simulink model "System_R2"  (R2018b)
settings: Solver=VariableStepAuto  StartTime=0.0  StopTime=5  RelTol=1e-3
libraries: dspsrcs4 x2, simulink x2
settings Model: Creator=Whtest  LastModifiedBy=Whtest

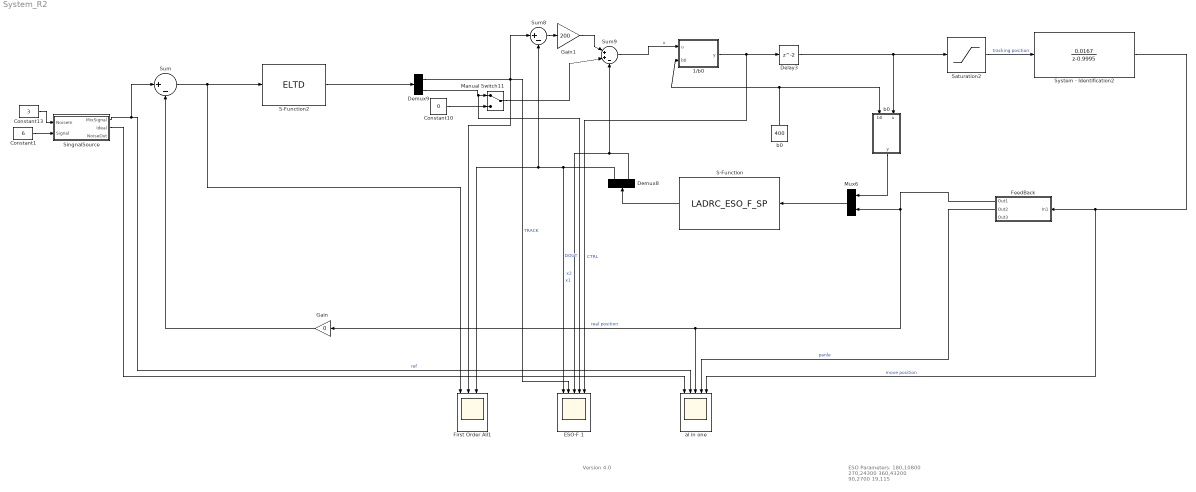
== system System_R2 ==
  note: ESO Parameters:
      | 180,10800
      | 270,24300
      | 360,43200
      | 90,2700
      | 19,115
  note: Version 4.0
  " b0" : MATLAB Function  TreatAsAtomicUnit=on
  1/b0 : MATLAB Function  TreatAsAtomicUnit=on
  Constant1 : Constant  Value=6
  Constant10 : Constant  Value=0
  Constant13 : Constant  Value=3
  Delay3 : Delay
  Demux8 : Demux  Outputs=2
  Demux9 : Demux  Outputs=2
  ESO-F 1 : Scope  NumInputPorts=5
  FeedBack : Subsystem
  First Order All1 : Scope  NumInputPorts=4
  Gain : Gain  Gain=0
  Gain1 : Gain  Gain=200
  Manual Switch11 : ManualSwitch
  Mux6 : Mux  Inputs=2
  S-Function : S-Function  FunctionName=LADRC_ESO_F_SP  Parameters=124  SFunctionDeploymentMode=off  EnableBusSupport=off
  S-Function2 : S-Function  FunctionName=ELTD  Parameters=1,6,10  SFunctionDeploymentMode=off  EnableBusSupport=off
  Saturation2 : Saturate  UpperLimit=1e5  LowerLimit=-1e5
  SingnalSource : Subsystem
  Sum : Sum  Inputs=|+-
  Sum8 : Sum  Inputs=|+-
  Sum9 : Sum  Inputs=|++-
  System - Identification2 : DiscreteTransferFcn  Numerator="[ 0    0.0167]"  Denominator="[1.0000   -0.9995]"
  al in one : Scope  NumInputPorts=5
  "b0 " : Constant  Value=400
  wires:
  " b0"/1(y) -> Mux6/1
  Demux8/2 -> ESO-F 1/3, Sum9/3  "x2"
  Sum8/1 -> Gain1/1
  1/b0/1(y) -> ESO-F 1/5, Delay3/1  "CTRL"
  Demux8/1 -> First Order All1/3, Sum8/2, ESO-F 1/1  "x1"
  Demux9/1 -> ESO-F 1/2, First Order All1/2, Sum8/1  "TRACK"
  Constant10/1 -> Manual Switch11/2
  Gain1/1 -> Sum9/1
  Saturation2/1 -> System - Identification2/1  "tracking position"
  Demux9/2 -> ESO-F 1/4, Manual Switch11/1  "DOUT"
  Mux6/1 -> S-Function/1
  Delay3/1 -> Saturation2/1, " b0"/2(u)
  Sum9/1 -> 1/b0/1(u)  "u"
  S-Function/1 -> Demux8/1
  Constant13/1 -> SingnalSource/1(NoiseIn)
  Constant1/1 -> SingnalSource/2(Signal)
  SingnalSource/1(MixSignal) -> al in one/2, Sum/1  "ref"
  Sum/1 -> First Order All1/1, S-Function2/1
  System - Identification2/1 -> al in one/5, FeedBack/1(In1)  "move position"
  S-Function2/1 -> Demux9/1
  SingnalSource/2(Ideal) -> al in one/1
  Gain/1 -> Sum/2
  "b0 "/1 -> 1/b0/2(b0), " b0"/1(b0)
  FeedBack/1(Out1) -> Gain/1, al in one/3, Mux6/2  "real position"
  FeedBack/2(Out2) -> al in one/4  "panle"
  Manual Switch11/1 -> Sum9/2

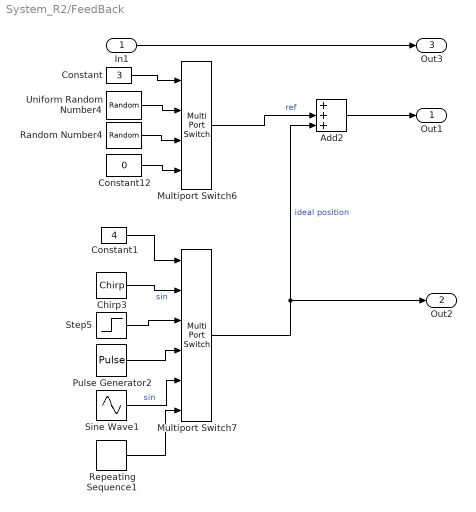
== system System_R2/FeedBack ==
  In1 : Inport
  Add2 : Sum  Inputs=+++
  Chirp3 : dspsrcs4/Chirp  sweep=Linear  mode=Unidirectional  f0=0  f1=10  t1=5  Tsweep=5  phase=0  Ts=0.001  spf=1  datatype=Double  OutputFrames=off
      settings: SourceProductName=DSP System Toolbox
  Constant : Constant  Value=3
  Constant1 : Constant  Value=4
  Constant12 : Constant  Value=0
  Multiport Switch6 : MultiPortSwitch
  Multiport Switch7 : MultiPortSwitch  Inputs=5
  Pulse Generator2 : DiscretePulseGenerator  PulseType=Time based  PulseWidth=50
  Random Number4 : RandomNumber  Variance=0.01  SampleTime=0.001
  Repeating Sequence1 : simulink/Sources/Repeating Sequence  rep_seq_t=[0 2 4 ]  rep_seq_y=[0 20 0 ]
  Sine Wave1 : Sin  Frequency=31.4  Phase=1*pi  SampleTime=0
  Step5 : Step  Time=0  After=0  SampleTime=5e-4
  Uniform Random Number4 : UniformRandomNumber  Minimum=-0.1  Maximum=0.1  SampleTime=0.001
  Out1 : Outport
  Out2 : Outport  Port=2
  Out3 : Outport  Port=3
  wires:
  In1/1 -> Out3/1
  Random Number4/1 -> Multiport Switch6/3
  Constant12/1 -> Multiport Switch6/4
  Uniform Random Number4/1 -> Multiport Switch6/2
  Constant/1 -> Multiport Switch6/1
  Sine Wave1/1 -> Multiport Switch7/5  "sin"
  Step5/1 -> Multiport Switch7/3
  Pulse Generator2/1 -> Multiport Switch7/4
  Constant1/1 -> Multiport Switch7/1
  Repeating Sequence1/1 -> Multiport Switch7/6
  Chirp3/1 -> Multiport Switch7/2  "sin"
  Multiport Switch7/1 -> Add2/3, Out2/1  "ideal position"
  Multiport Switch6/1 -> Add2/2  "ref"
  Add2/1 -> Out1/1

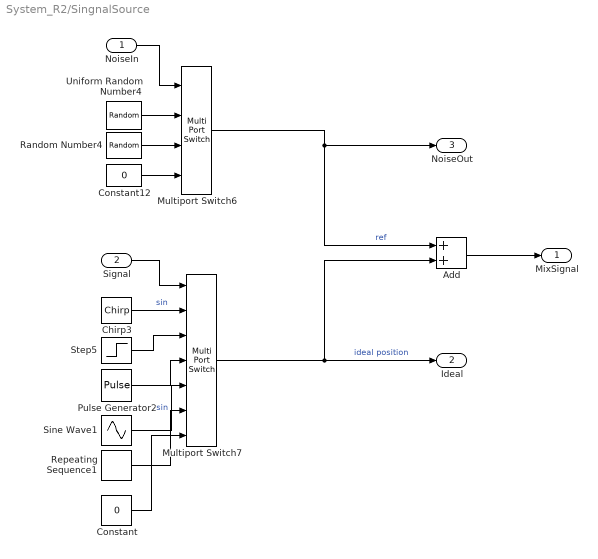
== system System_R2/SingnalSource ==
  NoiseIn : Inport
  Signal : Inport  Port=2
  Add : Sum
  Chirp3 : dspsrcs4/Chirp  sweep=Linear  mode=Unidirectional  f0=5  f1=5  t1=5  Tsweep=5  phase=1.5*pi  Ts=0.001  spf=1  datatype=Double  OutputFrames=off
      settings: SourceProductName=DSP System Toolbox
  Constant : Constant  Value=0
  Constant12 : Constant  Value=0
  Multiport Switch6 : MultiPortSwitch
  Multiport Switch7 : MultiPortSwitch  Inputs=6
  Pulse Generator2 : DiscretePulseGenerator  PulseType=Time based  PulseWidth=50
  Random Number4 : RandomNumber  Variance=0.01  SampleTime=0.001
  Repeating Sequence1 : simulink/Sources/Repeating Sequence  rep_seq_t=[0 2 4 ]  rep_seq_y=[0 20 0 ]
  Sine Wave1 : Sin  Amplitude=2000  Frequency=6.28  SampleTime=0
  Step5 : Step  Time=0.5  SampleTime=5e-4
  Uniform Random Number4 : UniformRandomNumber  Minimum=-0.1  Maximum=0.1  SampleTime=0.001
  MixSignal : Outport
  Ideal : Outport  Port=2
  NoiseOut : Outport  Port=3
  wires:
  Uniform Random Number4/1 -> Multiport Switch6/2
  Constant12/1 -> Multiport Switch6/4
  NoiseIn/1 -> Multiport Switch6/1
  Random Number4/1 -> Multiport Switch6/3
  Multiport Switch6/1 -> NoiseOut/1, Add/1  "ref"
  Sine Wave1/1 -> Multiport Switch7/5  "sin"
  Multiport Switch7/1 -> Add/2, Ideal/1  "ideal position"
  Repeating Sequence1/1 -> Multiport Switch7/6
  Step5/1 -> Multiport Switch7/3
  Chirp3/1 -> Multiport Switch7/2  "sin"
  Pulse Generator2/1 -> Multiport Switch7/4
  Signal/1 -> Multiport Switch7/1
  Add/1 -> MixSignal/1
  Constant/1 -> Multiport Switch7/7

== matlab function System_R2/ b0 ==
  data: b0 input; y output; u input
function y = fcn(b0,u)
y = b0.*u;

== matlab function System_R2/1//b0 ==
  data: u input; b0 input; y output
function y = fcn(u,b0)
y = u./b0;
